simulink model "Decentralized_Controller"  (R2023a)
settings: Solver=VariableStepAuto  StartTime=0.0  StopTime=10.0  RelTol=1e-3
libraries: dspinverses x1, DaVinci_LibDynamical x1
settings Model: Creator=afons  LastModifiedBy=afons

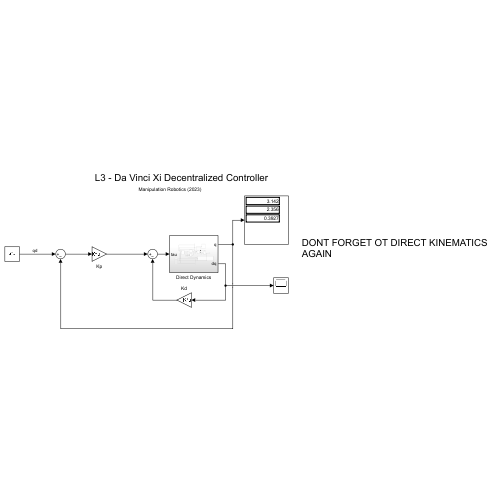
[thumbnail: Simulink's stored preview of the top-level diagram]
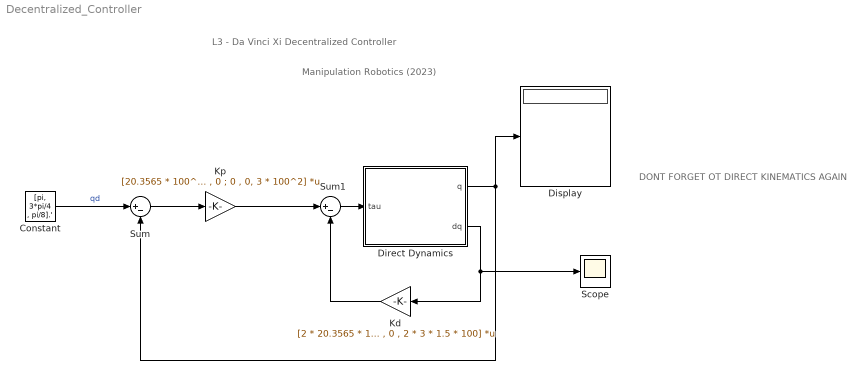
== system Decentralized_Controller ==
  note: Manipulation Robotics (2023)
  note: L3 - Da Vinci Xi Decentralized Controller
  note: DONT FORGET OT DIRECT KINEMATICS AGAIN
  Constant : Constant  Value=[pi, 3*pi/4 , pi/8].'  VectorParams1D=off
  Direct Dynamics : Subsystem
  Display : Display
  Kd : Gain  Gain=[2 * 20.3565 * 1.5 * 100 , 0 , 0 ; 0 , 2 * 2.0604 * 1.5 * 100,0 ; 0 , 0 , 2 * 3 * 1.5 * 100]  Multiplication=Matrix(K*u)
  Kp : Gain  Gain=[20.3565 * 100^2 , 0 , 0 ; 0 , 2.0604 * 100^2 , 0 ; 0 , 0, 3 * 100^2]  Multiplication=Matrix(K*u)
  Scope : Scope
  Sum : Sum  Inputs=|+-
  Sum1 : Sum  Inputs=|+-
  wires:
  Constant/1 -> Sum/1  "qd"
  Sum1/1 -> Direct Dynamics/1(tau)
  Direct Dynamics/1(q) -> Display/1, Sum/2
  Sum/1 -> Kp/1
  Kp/1 -> Sum1/1
  Direct Dynamics/2(dq) -> Scope/1, Kd/1
  Kd/1 -> Sum1/2

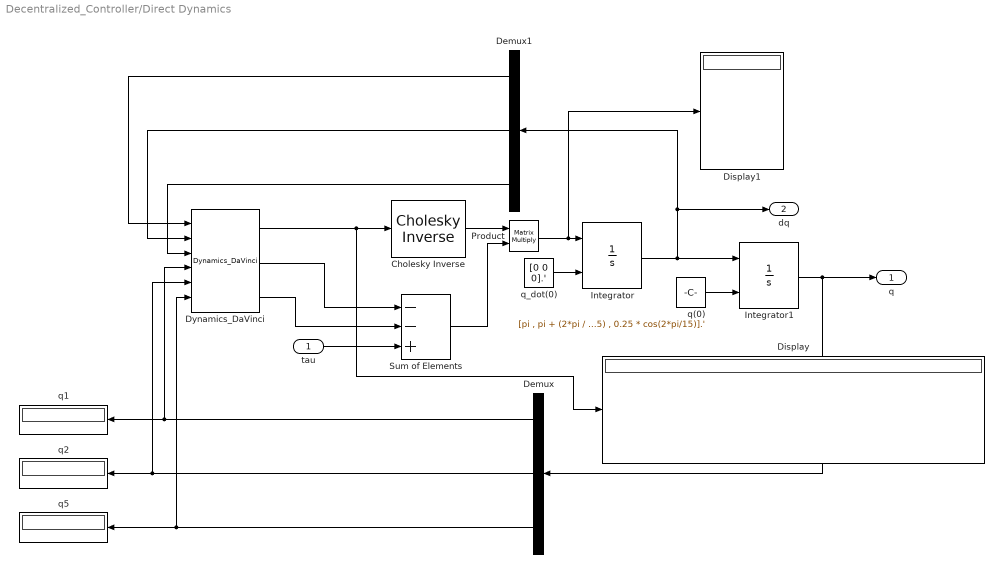
== system Decentralized_Controller/Direct Dynamics ==
  tau : Inport
  Cholesky Inverse : dspinverses/Cholesky Inverse  errmode=Warning
  Demux : Demux  Outputs=3
  Demux1 : Demux  Outputs=3
  Display : Display
  Display1 : Display
  Dynamics_DaVinci : DaVinci_LibDynamical/Dynamics_DaVinci  SystemSampleTime=-1  VariantActivationTime=update diagram  Latency=0  AutoFrameSizeCalculation=off
      settings: LibrarySourceBlock=|
      | simulink/User-Defined
      | Functions/MATLAB Function
  Integrator : Integrator  InitialConditionSource=external
  Integrator1 : Integrator  InitialConditionSource=external
  Product : Product  Multiplication=Matrix(*)
  Sum of Elements : Sum  Inputs=--+
  q(0) : Constant  Value=[pi , pi + (2*pi / 15) , 0.25 * cos(2*pi/15)].'
  q1 : Display
  q2 : Display
  q5 : Display
  q_dot(0) : Constant  Value=[0 0 0].'
  q : Outport
  dq : Outport  Port=2
  wires:
  Demux1/3 -> Dynamics_DaVinci/3
  Demux1/1 -> Dynamics_DaVinci/1
  Dynamics_DaVinci/1 -> Cholesky Inverse/1, Display/1
  Integrator/1 -> dq/1, Demux1/1, Integrator1/1
  Demux1/2 -> Dynamics_DaVinci/2
  q(0)/1 -> Integrator1/2
  Demux/2 -> Dynamics_DaVinci/5, q2/1
  q_dot(0)/1 -> Integrator/2
  Sum of Elements/1 -> Product/2
  Demux/1 -> Dynamics_DaVinci/4, q1/1
  Demux/3 -> Dynamics_DaVinci/6, q5/1
  Cholesky Inverse/1 -> Product/1
  Integrator1/1 -> q/1, Demux/1
  tau/1 -> Sum of Elements/3
  Dynamics_DaVinci/3 -> Sum of Elements/2
  Product/1 -> Display1/1, Integrator/1
  Dynamics_DaVinci/2 -> Sum of Elements/1
